simulink model "double_vitrage_1"  (R2019b)
settings: Solver=VariableStepAuto  StartTime=0.0  StopTime=24*3600  RelTol=1e-3
values from neighbouring files (symbols this model uses):
  ea = 10    [Parametres_double_vitrage.m]
  ev = 8    [Parametres_double_vitrage.m]
  T_ext = 10    [Parametres_double_vitrage.m]
  T_int = 20    [Parametres_double_vitrage.m]
libraries: fl_lib x29, nesl_utility x6
settings Model: Creator=Ivan  LastModifiedBy=ivanl
settings DataIOCC: ReturnWorkspaceOutputs=off
settings DebuggingCC: ArithmeticOperatorsInVariantConditions=warning
settings SFSimCC: SimUseLocalCustomCode=off  CustomCodeUndefinedFunction=UseInterfaceOnly
settings RTWCC: RTWUseLocalCustomCode=off
settings CodeAppCC: StateflowObjectComments=on
settings SimscapeCC: SimscapeNormalizeSystem=off  SimscapeLogType=all  SimscapeLogLimitData=off

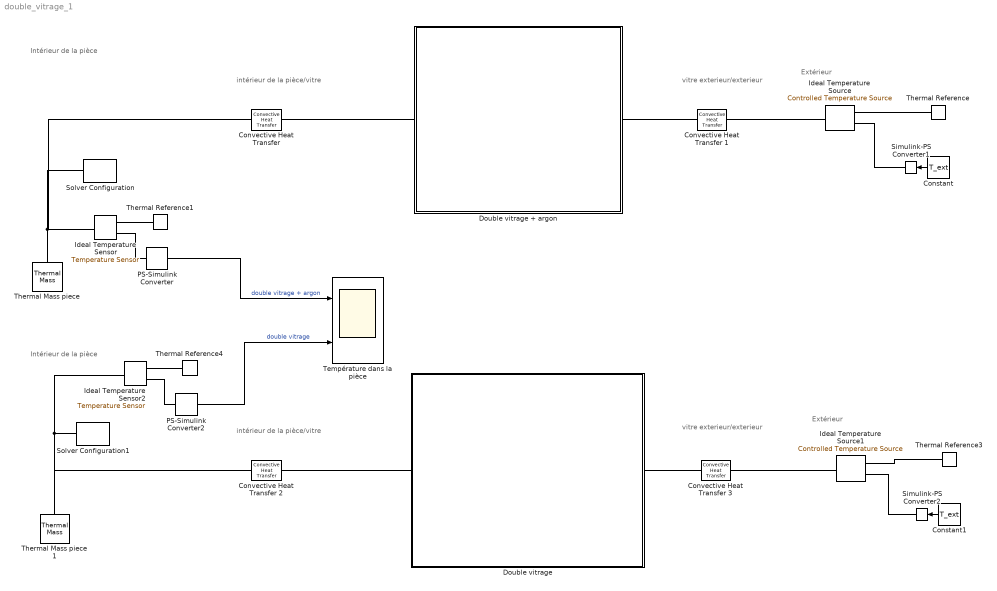
== system double_vitrage_1 ==
  note: Extérieur
  note: Intérieur de la pièce
  note: intérieur de la
      | pièce/vitre
  note: vitre exterieur/exterieur
  note: Intérieur de la pièce
  note: intérieur de la
      | pièce/vitre
  note: Extérieur
  note: vitre exterieur/exterieur
  Constant : Constant  Value=T_ext
  Constant1 : Constant  Value=T_ext
  "Convective Heat Transfer " : fl_lib/Thermal/Thermal Elements/Convective Heat Transfer  area=A m^2  heat_tr_coeff=ksi W/(m^2 * K)  T_specify=off  T_priority=None  T=20 degC  T_nominal_specify=off  T_nominal_unit=K  T_nominal_value=1  Q_specify=off  Q_priority=None  Q=0 J/s  Q_nominal_specify=off  Q_nominal_unit=J/s  Q_nominal_value=1
  Convective Heat Transfer 1 : fl_lib/Thermal/Thermal Elements/Convective Heat Transfer  area=A m^2  heat_tr_coeff=kse W/(m^2 * K)  T_specify=off  T_priority=None  T=0 K  T_nominal_specify=off  T_nominal_unit=K  T_nominal_value=1  Q_specify=off  Q_priority=None  Q=0 J/s  Q_nominal_specify=off  Q_nominal_unit=J/s  Q_nominal_value=1
  Convective Heat Transfer 2 : fl_lib/Thermal/Thermal Elements/Convective Heat Transfer  area=A m^2  heat_tr_coeff=ksi W/(m^2 * K)  T_specify=off  T_priority=None  T=20 degC  T_nominal_specify=off  T_nominal_unit=K  T_nominal_value=1  Q_specify=off  Q_priority=None  Q=0 J/s  Q_nominal_specify=off  Q_nominal_unit=J/s  Q_nominal_value=1
  Convective Heat Transfer 3 : fl_lib/Thermal/Thermal Elements/Convective Heat Transfer  area=A m^2  heat_tr_coeff=kse W/(m^2 * K)  T_specify=off  T_priority=None  T=0 K  T_nominal_specify=off  T_nominal_unit=K  T_nominal_value=1  Q_specify=off  Q_priority=None  Q=0 J/s  Q_nominal_specify=off  Q_nominal_unit=J/s  Q_nominal_value=1
  Double vitrage : Subsystem
      mask Display: image(imread('image_double_vitrage.jpg'))
  Double vitrage + argon : Subsystem
      mask Display: image(imread('image_double_vitrage_argon.jpg'))
  Ideal Temperature Sensor : fl_lib/Thermal/Thermal Sensors/Temperature Sensor
  Ideal Temperature Sensor2 : fl_lib/Thermal/Thermal Sensors/Temperature Sensor
  Ideal Temperature Source : fl_lib/Thermal/Thermal Sources/Controlled Temperature Source
      settings: SourceProductName=Simscape
  Ideal Temperature Source1 : fl_lib/Thermal/Thermal Sources/Controlled Temperature Source
      settings: SourceProductName=Simscape
  PS-Simulink Converter : nesl_utility/PS-Simulink Converter  PhysicalDomain=network_engine_domain  SubClassName=ps_output  LeftPortType=input  RightPortType=output  PseudoPeriodic=off  Frequencies=[]  Unit=degC  AffineConversion=on
  PS-Simulink Converter2 : nesl_utility/PS-Simulink Converter  PhysicalDomain=network_engine_domain  SubClassName=ps_output  LeftPortType=input  RightPortType=output  PseudoPeriodic=off  Frequencies=[]  Unit=degC  AffineConversion=on
  Simulink-PS Converter1 : nesl_utility/Simulink-PS Converter  PhysicalDomain=network_engine_domain  SubClassName=ps_input  LeftPortType=input  RightPortType=output  PseudoPeriodic=off  Frequencies=[]  NoiseDistribution=none  NoiseParameters=[]  Unit=degC  AffineConversion=on  FilteringAndDerivatives=provide  SimscapeFilterOrder=1  InputFilterTimeConstant=0.001  UdotUserProvided=0
  Simulink-PS Converter2 : nesl_utility/Simulink-PS Converter  PhysicalDomain=network_engine_domain  SubClassName=ps_input  LeftPortType=input  RightPortType=output  PseudoPeriodic=off  Frequencies=[]  NoiseDistribution=none  NoiseParameters=[]  Unit=degC  AffineConversion=on  FilteringAndDerivatives=provide  SimscapeFilterOrder=1  InputFilterTimeConstant=0.001  UdotUserProvided=0
  Solver Configuration : nesl_utility/Solver Configuration  PhysicalDomain=network_engine_domain  SubClassName=solver  LeftPortType=input  RightPortType=generic  Tones=[]  Harmonics=[]  SimulateNoise=off  Profile=off  UseLocalSampling=off  EnableSwitchedLinearOptims=on  FrequencyDomain=off  UseCCode=off  RelTol=0.001  AbsTol=1e-06  MinStep=1e-09  ToWorkspace=off  RevertToSquareIcSolve=off  NumHomotopyIterations=100  PhasorMode=off  PhasorModeNumHarmonics=1  DoDC=off  ResidualTolerance=1e-09  UseLocalSolver=off  LocalSolverChoice=NE_BACKWARD_EULER_ADVANCER  LocalSolverSampleTime=0.001  DoFixedCost=off  MaxNonlinIter=3  MaxModeIter=2  LinearAlgebra=Sparse  EquationFormulation=NE_TIME_EF  DelaysMemoryBudget=1024  AutomaticFiltering=on  FilteringTimeConstant=0.001  PartitionStorageMethod=AS_NEEDED  PartitionMemoryBudget=1024  PartitionMethod=FAST
  Solver Configuration1 : nesl_utility/Solver Configuration  PhysicalDomain=network_engine_domain  SubClassName=solver  LeftPortType=input  RightPortType=generic  Tones=[]  Harmonics=[]  SimulateNoise=off  Profile=off  UseLocalSampling=off  EnableSwitchedLinearOptims=on  FrequencyDomain=off  UseCCode=off  RelTol=0.001  AbsTol=1e-06  MinStep=1e-09  ToWorkspace=off  RevertToSquareIcSolve=off  NumHomotopyIterations=100  PhasorMode=off  PhasorModeNumHarmonics=1  DoDC=off  ResidualTolerance=1e-09  UseLocalSolver=off  LocalSolverChoice=NE_BACKWARD_EULER_ADVANCER  LocalSolverSampleTime=0.001  DoFixedCost=off  MaxNonlinIter=3  MaxModeIter=2  LinearAlgebra=Sparse  EquationFormulation=NE_TIME_EF  DelaysMemoryBudget=1024  AutomaticFiltering=on  FilteringTimeConstant=0.001  PartitionStorageMethod=AS_NEEDED  PartitionMemoryBudget=1024  PartitionMethod=FAST
  Température dans la pièce : Scope  NumInputPorts=2
  "Thermal Mass piece " : fl_lib/Thermal/Thermal Elements/Thermal Mass  mass=Mair kg  sp_heat=cair J/kg/K  T_specify=on  T_priority=High  T=20 degC  T_nominal_specify=off  T_nominal_unit=K  T_nominal_value=1  Q_specify=off  Q_priority=None  Q=0 J/s  Q_nominal_specify=off  Q_nominal_unit=J/s  Q_nominal_value=1
  Thermal Mass piece 1 : fl_lib/Thermal/Thermal Elements/Thermal Mass  mass=Mair kg  sp_heat=cair J/kg/K  T_specify=on  T_priority=High  T=20 degC  T_nominal_specify=off  T_nominal_unit=K  T_nominal_value=1  Q_specify=off  Q_priority=None  Q=0 J/s  Q_nominal_specify=off  Q_nominal_unit=J/s  Q_nominal_value=1
  Thermal Reference{,1,3..4} (4 alike) : fl_lib/Thermal/Thermal Elements/Thermal Reference
  wires:
  PS-Simulink Converter/1 -> Température dans la pièce/1  "double vitrage + argon"
  Constant/1 -> Simulink-PS Converter1/1
  Constant1/1 -> Simulink-PS Converter2/1
  PS-Simulink Converter2/1 -> Température dans la pièce/2  "double vitrage"
  connections:
  "Thermal Mass piece "/LConn1 -- "Convective Heat Transfer "/LConn1 -- Solver Configuration/RConn1 -- Ideal Temperature Sensor/LConn1
  Ideal Temperature Source/LConn1 -- Convective Heat Transfer 1/RConn1
  Simulink-PS Converter1/RConn1 -- Ideal Temperature Source/RConn1
  Thermal Reference/LConn1 -- Ideal Temperature Source/RConn2
  Thermal Reference1/LConn1 -- Ideal Temperature Sensor/RConn1
  PS-Simulink Converter/LConn1 -- Ideal Temperature Sensor/RConn2
  Solver Configuration1/RConn1 -- Convective Heat Transfer 2/LConn1 -- Thermal Mass piece 1/LConn1 -- Ideal Temperature Sensor2/LConn1
  Simulink-PS Converter2/RConn1 -- Ideal Temperature Source1/RConn1
  Ideal Temperature Source1/LConn1 -- Convective Heat Transfer 3/RConn1
  Thermal Reference3/LConn1 -- Ideal Temperature Source1/RConn2
  PS-Simulink Converter2/LConn1 -- Ideal Temperature Sensor2/RConn2
  Thermal Reference4/LConn1 -- Ideal Temperature Sensor2/RConn1
  "Convective Heat Transfer "/RConn1 -- Double vitrage + argon/LConn1
  Double vitrage + argon/RConn1 -- Convective Heat Transfer 1/LConn1
  Double vitrage/LConn1 -- Convective Heat Transfer 2/RConn1
  Double vitrage/RConn1 -- Convective Heat Transfer 3/LConn1

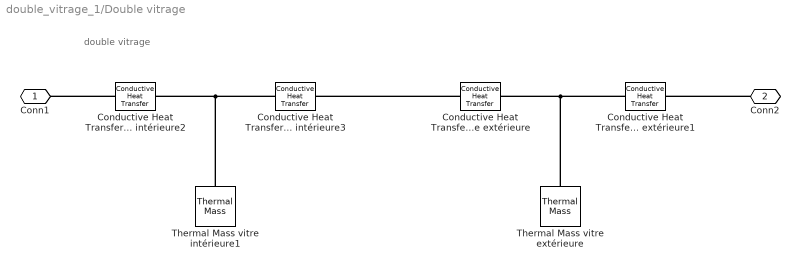
== system double_vitrage_1/Double vitrage ==
  note: double vitrage
  Conductive Heat Transfer demi-paroi vitre extérieure : fl_lib/Thermal/Thermal Elements/Conductive Heat Transfer  area=A m^2  thickness=ev/2 mm  th_cond=lam_v W/(m*K)  T_specify=off  T_priority=None  T=0 K  T_nominal_specify=off  T_nominal_unit=K  T_nominal_value=1  Q_specify=off  Q_priority=None  Q=0 J/s  Q_nominal_specify=off  Q_nominal_unit=J/s  Q_nominal_value=1
      settings: SourceProductName=Simscape
  Conductive Heat Transfer demi-paroi vitre extérieure1 : fl_lib/Thermal/Thermal Elements/Conductive Heat Transfer  area=A m^2  thickness=ev/2 mm  th_cond=lam_v W/(m*K)  T_specify=off  T_priority=None  T=0 K  T_nominal_specify=off  T_nominal_unit=K  T_nominal_value=1  Q_specify=off  Q_priority=None  Q=0 J/s  Q_nominal_specify=off  Q_nominal_unit=J/s  Q_nominal_value=1
      settings: SourceProductName=Simscape
  Conductive Heat Transfer demi-paroi vitre intérieure2 : fl_lib/Thermal/Thermal Elements/Conductive Heat Transfer  area=A m^2  thickness=ev/2 mm  th_cond=lam_v W/(m*K)  T_specify=off  T_priority=None  T=0 K  T_nominal_specify=off  T_nominal_unit=K  T_nominal_value=1  Q_specify=off  Q_priority=None  Q=0 J/s  Q_nominal_specify=off  Q_nominal_unit=J/s  Q_nominal_value=1
      settings: SourceProductName=Simscape
  Conductive Heat Transfer demi-paroi vitre intérieure3 : fl_lib/Thermal/Thermal Elements/Conductive Heat Transfer  area=A m^2  thickness=ev/2 mm  th_cond=lam_v W/(m*K)  T_specify=off  T_priority=None  T=0 K  T_nominal_specify=off  T_nominal_unit=K  T_nominal_value=1  Q_specify=off  Q_priority=None  Q=0 J/s  Q_nominal_specify=off  Q_nominal_unit=J/s  Q_nominal_value=1
      settings: SourceProductName=Simscape
  Thermal Mass vitre extérieure : fl_lib/Thermal/Thermal Elements/Thermal Mass  mass=Mv kg  sp_heat=cv J/kg/K  T_specify=on  T_priority=High  T=T_int degC  T_nominal_specify=off  T_nominal_unit=K  T_nominal_value=1  Q_specify=off  Q_priority=None  Q=0 J/s  Q_nominal_specify=off  Q_nominal_unit=J/s  Q_nominal_value=1
  Thermal Mass vitre intérieure1 : fl_lib/Thermal/Thermal Elements/Thermal Mass  mass=Mv kg  sp_heat=cv J/kg/K  T_specify=on  T_priority=High  T=T_int degC  T_nominal_specify=off  T_nominal_unit=K  T_nominal_value=1  Q_specify=off  Q_priority=None  Q=0 J/s  Q_nominal_specify=off  Q_nominal_unit=J/s  Q_nominal_value=1
  Conn1 : PMIOPort  Side=Left
  Conn2 : PMIOPort  Port=2  Side=Right
  connections:
  Conductive Heat Transfer demi-paroi vitre intérieure3/LConn1 -- Conductive Heat Transfer demi-paroi vitre intérieure2/RConn1 -- Thermal Mass vitre intérieure1/LConn1
  Conductive Heat Transfer demi-paroi vitre intérieure2/LConn1 -- Conn1/RConn1
  Conductive Heat Transfer demi-paroi vitre extérieure1/LConn1 -- Thermal Mass vitre extérieure/LConn1 -- Conductive Heat Transfer demi-paroi vitre extérieure/RConn1
  Conductive Heat Transfer demi-paroi vitre extérieure/LConn1 -- Conductive Heat Transfer demi-paroi vitre intérieure3/RConn1
  Conn2/RConn1 -- Conductive Heat Transfer demi-paroi vitre extérieure1/RConn1

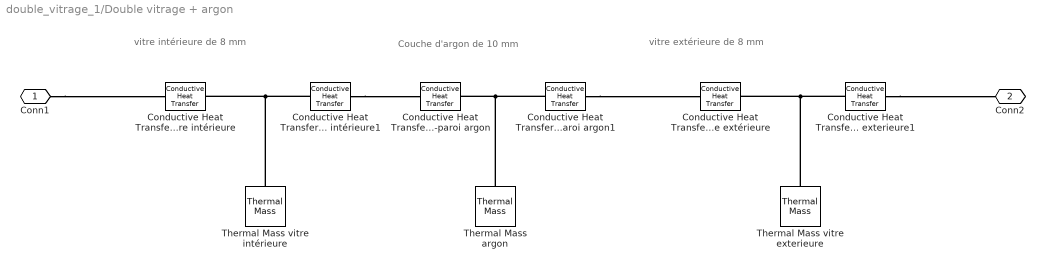
== system double_vitrage_1/Double vitrage + argon ==
  note: Couche d'argon de 10 mm
  note: vitre intérieure de 8 mm
  note: vitre extérieure de 8 mm
  Conductive Heat Transfer demi-paroi argon : fl_lib/Thermal/Thermal Elements/Conductive Heat Transfer  area=A m^2  thickness=ea/2 mm  th_cond=lam_a W/(m*K)  T_specify=off  T_priority=None  T=0 K  T_nominal_specify=off  T_nominal_unit=K  T_nominal_value=1  Q_specify=off  Q_priority=None  Q=0 J/s  Q_nominal_specify=off  Q_nominal_unit=J/s  Q_nominal_value=1
      settings: SourceProductName=Simscape
  Conductive Heat Transfer demi-paroi argon1 : fl_lib/Thermal/Thermal Elements/Conductive Heat Transfer  area=A m^2  thickness=ea/2 mm  th_cond=lam_a W/(m*K)  T_specify=off  T_priority=None  T=0 K  T_nominal_specify=off  T_nominal_unit=K  T_nominal_value=1  Q_specify=off  Q_priority=None  Q=0 J/s  Q_nominal_specify=off  Q_nominal_unit=J/s  Q_nominal_value=1
      settings: SourceProductName=Simscape
  Conductive Heat Transfer demi-paroi vitre exterieure1 : fl_lib/Thermal/Thermal Elements/Conductive Heat Transfer  area=A m^2  thickness=ev/2 mm  th_cond=lam_v W/(m*K)  T_specify=off  T_priority=None  T=0 K  T_nominal_specify=off  T_nominal_unit=K  T_nominal_value=1  Q_specify=off  Q_priority=None  Q=0 J/s  Q_nominal_specify=off  Q_nominal_unit=J/s  Q_nominal_value=1
      settings: SourceProductName=Simscape
  Conductive Heat Transfer demi-paroi vitre extérieure : fl_lib/Thermal/Thermal Elements/Conductive Heat Transfer  area=A m^2  thickness=ev/2 mm  th_cond=lam_v W/(m*K)  T_specify=off  T_priority=None  T=0 K  T_nominal_specify=off  T_nominal_unit=K  T_nominal_value=1  Q_specify=off  Q_priority=None  Q=0 J/s  Q_nominal_specify=off  Q_nominal_unit=J/s  Q_nominal_value=1
      settings: SourceProductName=Simscape
  Conductive Heat Transfer demi-paroi vitre intérieure : fl_lib/Thermal/Thermal Elements/Conductive Heat Transfer  area=A m^2  thickness=ev/2 mm  th_cond=lam_v W/(m*K)  T_specify=off  T_priority=None  T=0 K  T_nominal_specify=off  T_nominal_unit=K  T_nominal_value=1  Q_specify=off  Q_priority=None  Q=0 J/s  Q_nominal_specify=off  Q_nominal_unit=J/s  Q_nominal_value=1
      settings: SourceProductName=Simscape
  Conductive Heat Transfer demi-paroi vitre intérieure1 : fl_lib/Thermal/Thermal Elements/Conductive Heat Transfer  area=A m^2  thickness=ev/2 mm  th_cond=lam_v W/(m*K)  T_specify=off  T_priority=None  T=0 K  T_nominal_specify=off  T_nominal_unit=K  T_nominal_value=1  Q_specify=off  Q_priority=None  Q=0 J/s  Q_nominal_specify=off  Q_nominal_unit=J/s  Q_nominal_value=1
      settings: SourceProductName=Simscape
  Thermal Mass argon : fl_lib/Thermal/Thermal Elements/Thermal Mass  mass=Ma kg  sp_heat=ca J/kg/K  T_specify=on  T_priority=High  T=(T_int+T_ext)/2 degC  T_nominal_specify=off  T_nominal_unit=K  T_nominal_value=1  Q_specify=off  Q_priority=None  Q=0 J/s  Q_nominal_specify=off  Q_nominal_unit=J/s  Q_nominal_value=1
  Thermal Mass vitre exterieure : fl_lib/Thermal/Thermal Elements/Thermal Mass  mass=Mv kg  sp_heat=lam_v J/kg/K  T_specify=on  T_priority=High  T=T_ext degC  T_nominal_specify=off  T_nominal_unit=K  T_nominal_value=1  Q_specify=off  Q_priority=None  Q=0 J/s  Q_nominal_specify=off  Q_nominal_unit=J/s  Q_nominal_value=1
  Thermal Mass vitre intérieure : fl_lib/Thermal/Thermal Elements/Thermal Mass  mass=Mv kg  sp_heat=cv J/kg/K  T_specify=on  T_priority=High  T=T_int degC  T_nominal_specify=off  T_nominal_unit=K  T_nominal_value=1  Q_specify=off  Q_priority=None  Q=0 J/s  Q_nominal_specify=off  Q_nominal_unit=J/s  Q_nominal_value=1
  Conn1 : PMIOPort  Side=Left
  Conn2 : PMIOPort  Port=2  Side=Right
  connections:
  Thermal Mass vitre intérieure/LConn1 -- Conductive Heat Transfer demi-paroi vitre intérieure1/LConn1 -- Conductive Heat Transfer demi-paroi vitre intérieure/RConn1
  Conductive Heat Transfer demi-paroi argon1/RConn1 -- Conductive Heat Transfer demi-paroi vitre extérieure/LConn1
  Conductive Heat Transfer demi-paroi vitre exterieure1/LConn1 -- Thermal Mass vitre exterieure/LConn1 -- Conductive Heat Transfer demi-paroi vitre extérieure/RConn1
  Conductive Heat Transfer demi-paroi vitre exterieure1/RConn1 -- Conn2/RConn1
  Conn1/RConn1 -- Conductive Heat Transfer demi-paroi vitre intérieure/LConn1
  Conductive Heat Transfer demi-paroi vitre intérieure1/RConn1 -- Conductive Heat Transfer demi-paroi argon/LConn1
  Thermal Mass argon/LConn1 -- Conductive Heat Transfer demi-paroi argon1/LConn1 -- Conductive Heat Transfer demi-paroi argon/RConn1
